simulink model "Simulation_StateLinear_PostureReg"  (R2022b)
settings: Solver=FixedStepAuto  StartTime=0.0  StopTime=200  FixedStep=0.02  RelTol=1e-3
undefined symbols (not defined in the file): theta_des, theta_f, unicycle, x_des, x_f, y_des, y_f
libraries: simulink_extras x3, dspsigops x2
settings Model: Creator=Musta  LastModifiedBy=Musta

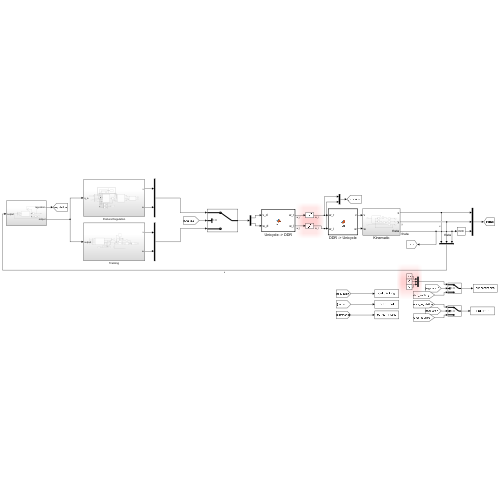
[thumbnail: Simulink's stored preview of the top-level diagram]
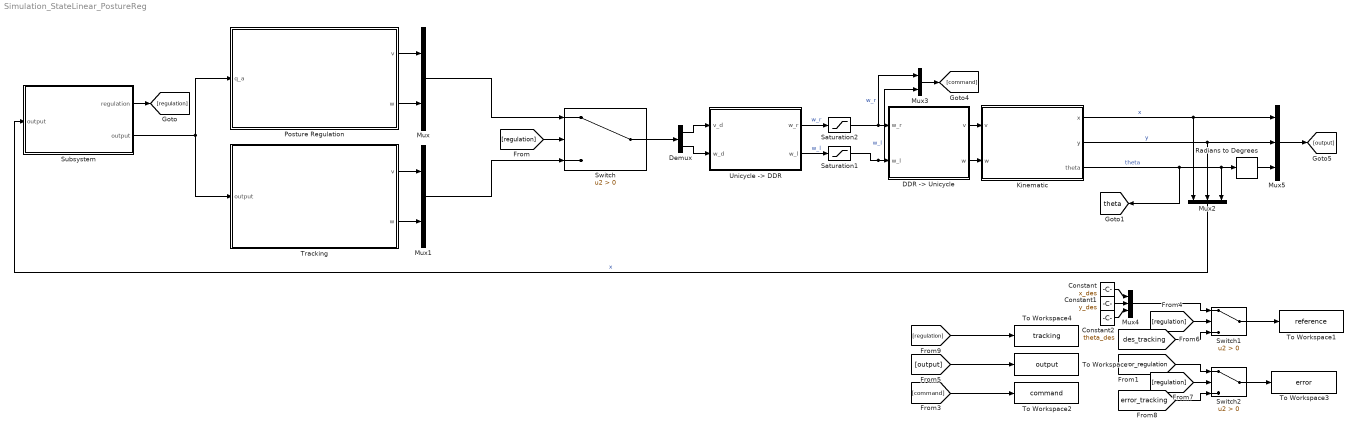
== system Simulation_StateLinear_PostureReg ==
  " DDR -> Unicycle " : MATLAB Function  TreatAsAtomicUnit=on
  Constant : Constant  Value=x_des
  Constant1 : Constant  Value=y_des
  Constant2 : Constant  Value=theta_des
  Demux : Demux  Outputs=2
  Kinematic : Subsystem
  Mux : Mux  Inputs=2
  Mux1 : Mux  Inputs=2
  Mux2 : Mux  Inputs=3
  Mux3 : Mux  Inputs=2
  Mux4 : Mux  Inputs=3
  Mux5 : Mux  Inputs=3
  Posture Regulation : Subsystem
  Radians to Degrees : simulink_extras/Transformations/Radians to Degrees
  Saturation1 : Saturate  UpperLimit=unicycle.omegaWheelMax  LowerLimit=unicycle.omegaWheelMin
  Saturation2 : Saturate  UpperLimit=unicycle.omegaWheelMax  LowerLimit=unicycle.omegaWheelMin
  Subsystem : Subsystem
  Switch : Switch  Criteria=u2 > Threshold  SaturateOnIntegerOverflow=off  InputSameDT=off
  Switch1 : Switch  Criteria=u2 > Threshold  SaturateOnIntegerOverflow=off  InputSameDT=off
  Switch2 : Switch  Criteria=u2 > Threshold  SaturateOnIntegerOverflow=off  InputSameDT=off
  To Workspace : ToWorkspace  VariableName=output  SaveFormat=Structure With Time  SampleTime=-1
  To Workspace1 : ToWorkspace  VariableName=reference  SaveFormat=Structure With Time  SampleTime=-1
  To Workspace2 : ToWorkspace  VariableName=command  SaveFormat=Structure With Time  SampleTime=-1
  To Workspace3 : ToWorkspace  VariableName=error  SaveFormat=Structure With Time  SampleTime=-1
  To Workspace4 : ToWorkspace  VariableName=tracking  SaveFormat=Structure With Time  SampleTime=-1
  Tracking : Subsystem
  "Unicycle -> DDR" : MATLAB Function  TreatAsAtomicUnit=on
  tag scope: theta=global
  wires:
  [error_regulation] -> Switch2/1
  [regulation] -> Switch2/2
  Switch1/1 -> To Workspace1/1
  Subsystem/2(output) -> Posture Regulation/1(q_a), Tracking/1(output)
  Switch/1 -> Demux/1
  Mux1/1 -> Switch/3
  Tracking/2(w) -> Mux1/2
  Mux2/1 -> Subsystem/1("output ")  "x"
  [regulation] -> Switch/2
  [command] -> To Workspace2/1
  Posture Regulation/2(w) -> Mux/2
  Subsystem/1(regulation) -> [regulation]
  [error_tracking] -> Switch2/3
  Saturation1/1 -> Mux3/2, " DDR -> Unicycle "/2(w_l)  "w_l"
  "Unicycle -> DDR"/2(w_l) -> Saturation1/1  "w_l"
  Demux/1 -> "Unicycle -> DDR"/1(v_d)
  Posture Regulation/1(v) -> Mux/1
  Tracking/1(v) -> Mux1/1
  Mux/1 -> Switch/1
  [output] -> To Workspace/1
  Saturation2/1 -> Mux3/1, " DDR -> Unicycle "/1(w_r)  "w_r"
  Switch2/1 -> To Workspace3/1
  "Unicycle -> DDR"/1(w_r) -> Saturation2/1  "w_r"
  Demux/2 -> "Unicycle -> DDR"/2(w_d)
  Kinematic/2(y) -> Mux2/2, Mux5/2  "y"
  " DDR -> Unicycle "/1(v) -> Kinematic/1(v)
  Radians to Degrees/1 -> Mux5/3
  " DDR -> Unicycle "/2(w) -> Kinematic/2(w)
  Mux5/1 -> [output]
  Kinematic/3(theta) -> [theta], Mux2/3, Radians to Degrees/1  "theta"
  Kinematic/1(x) -> Mux2/1, Mux5/1  "x"
  Mux3/1 -> [command]
  [regulation] -> To Workspace4/1
  Mux4/1 -> Switch1/1
  [regulation] -> Switch1/2
  [des_tracking] -> Switch1/3
  Constant1/1 -> Mux4/2
  Constant/1 -> Mux4/1
  Constant2/1 -> Mux4/3

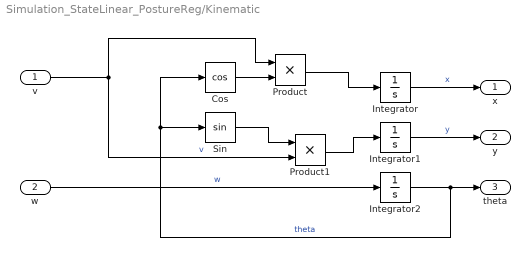
== system Simulation_StateLinear_PostureReg/Kinematic ==
  v : Inport
  w : Inport  Port=2
  Cos : Trigonometry  Operator=cos
  Integrator : Integrator  InitialCondition=unicycle.ic.x
  Integrator1 : Integrator  InitialCondition=unicycle.ic.y
  Integrator2 : Integrator  InitialCondition=unicycle.ic.theta
  Product : Product
  Product1 : Product
  Sin : Trigonometry
  x : Outport
  y : Outport  Port=2
  theta : Outport  Port=3
  wires:
  w/1 -> Integrator2/1  "w"
  Product/1 -> Integrator/1
  v/1 -> Product/1, Product1/2  "v"
  Cos/1 -> Product/2
  Integrator1/1 -> y/1  "y"
  Integrator/1 -> x/1  "x"
  Integrator2/1 -> Cos/1, Sin/1, theta/1  "theta"
  Product1/1 -> Integrator1/1
  Sin/1 -> Product1/1

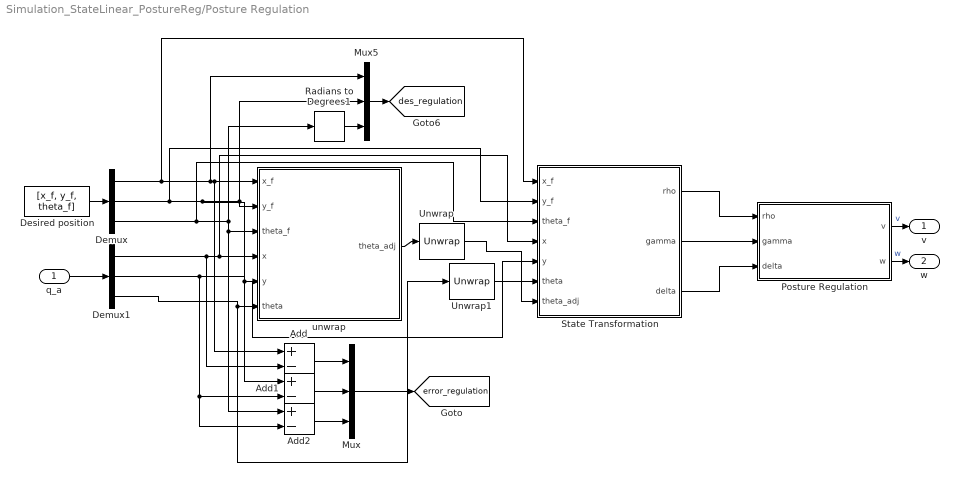
== system Simulation_StateLinear_PostureReg/Posture Regulation ==
  q_a : Inport
  Add : Sum  Inputs=+-
  Add1 : Sum  Inputs=+-
  Add2 : Sum  Inputs=+-
  Demux : Demux  Outputs=3
  Demux1 : Demux  Outputs=3
  Desired position : Constant  Value=[x_f, y_f, theta_f]
  Mux : Mux  Inputs=3
  Mux5 : Mux  Inputs=3
  Posture Regulation : MATLAB Function  TreatAsAtomicUnit=on
  Radians to Degrees1 : simulink_extras/Transformations/Radians to Degrees
  State Transformation : MATLAB Function  TreatAsAtomicUnit=on
  Unwrap : dspsigops/Unwrap  tol=pi  InputProcessing=Columns as channels (frame based)  running=off
  Unwrap1 : dspsigops/Unwrap  tol=pi  InputProcessing=Columns as channels (frame based)  running=off
  unwrap : MATLAB Function  TreatAsAtomicUnit=on
  v : Outport
  w : Outport  Port=2
  tag scope: des_regulation=global, error_regulation=global
  wires:
  Posture Regulation/1(v) -> v/1  "v"
  Radians to Degrees1/1 -> Mux5/3
  Posture Regulation/2(w) -> w/1  "w"
  Mux5/1 -> [des_regulation]
  Desired position/1 -> Demux/1
  Demux/3 -> State Transformation/3(theta_f), Add2/1, unwrap/3(theta_f), Radians to Degrees1/1
  Demux/2 -> State Transformation/2(y_f), Add1/1, Mux5/2, unwrap/2(y_f)
  Demux/1 -> State Transformation/1(x_f), Mux5/1, Add/1, unwrap/1(x_f)
  Demux1/1 -> Add/2, State Transformation/4(x), unwrap/4(x)
  Demux1/2 -> Add2/2, Add1/2, State Transformation/5(y), unwrap/5(y)
  Demux1/3 -> Unwrap1/1, unwrap/6(theta)
  q_a/1 -> Demux1/1
  Add/1 -> Mux/1
  Add1/1 -> Mux/2
  Add2/1 -> Mux/3
  Mux/1 -> [error_regulation]
  State Transformation/2(gamma) -> Posture Regulation/2(gamma)
  State Transformation/1(rho) -> Posture Regulation/1(rho)
  State Transformation/3(delta) -> Posture Regulation/3(delta)
  unwrap/1(theta_adj) -> Unwrap/1
  Unwrap/1 -> State Transformation/7(theta_adj)
  Unwrap1/1 -> State Transformation/6(theta)

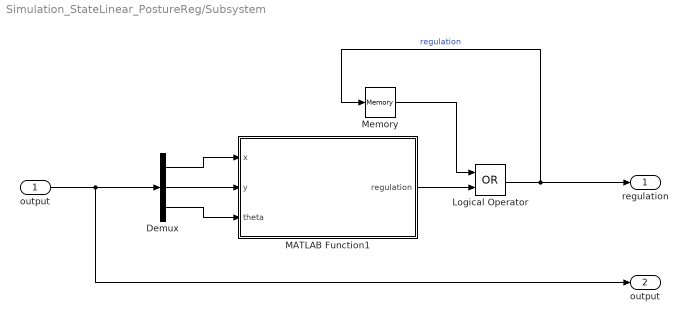
== system Simulation_StateLinear_PostureReg/Subsystem ==
  "output " : Inport
  Demux : Demux  Outputs=3
  Logical Operator : Logic  Operator=OR  AllPortsSameDT=off  OutDataTypeStr=boolean
  MATLAB Function1 : MATLAB Function  TreatAsAtomicUnit=on
  Memory : Memory
  regulation : Outport
  output : Outport  Port=2
  wires:
  Memory/1 -> Logical Operator/1
  Logical Operator/1 -> regulation/1, Memory/1  "regulation"
  MATLAB Function1/1(regulation) -> Logical Operator/2
  "output "/1 -> output/1, Demux/1
  Demux/3 -> MATLAB Function1/3(theta)
  Demux/2 -> MATLAB Function1/2(y)
  Demux/1 -> MATLAB Function1/1(x)

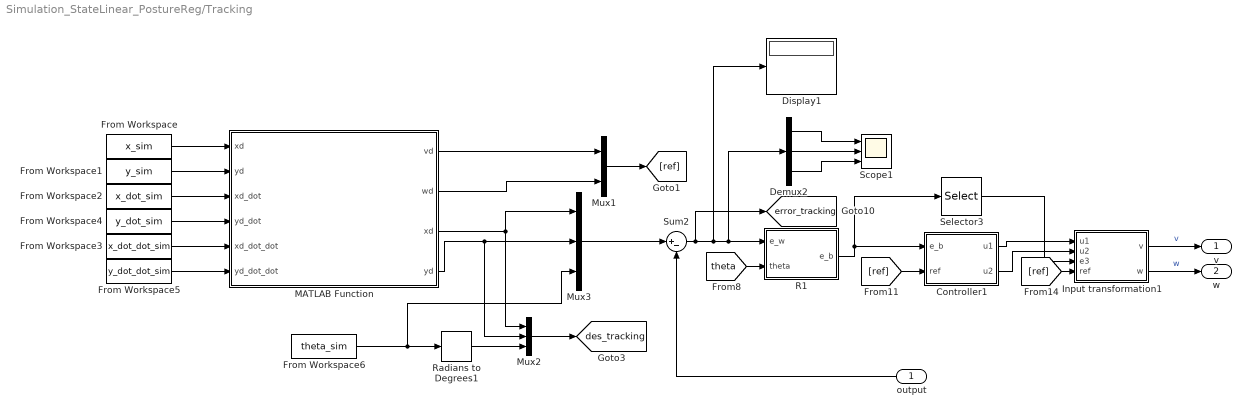
== system Simulation_StateLinear_PostureReg/Tracking ==
  output : Inport
  Controller1 : MATLAB Function  TreatAsAtomicUnit=on
  Demux2 : Demux  Outputs=3
  Display1 : Display
  From Workspace : FromWorkspace  VariableName=x_sim
  From Workspace1 : FromWorkspace  VariableName=y_sim
  From Workspace2 : FromWorkspace  VariableName=x_dot_sim
  From Workspace3 : FromWorkspace  VariableName=x_dot_dot_sim
  From Workspace4 : FromWorkspace  VariableName=y_dot_sim
  From Workspace5 : FromWorkspace  VariableName=y_dot_dot_sim
  From Workspace6 : FromWorkspace  VariableName=theta_sim
  Input transformation1 : MATLAB Function  TreatAsAtomicUnit=on
  MATLAB Function : MATLAB Function  TreatAsAtomicUnit=on
  Mux1 : Mux  Inputs=2
  Mux2 : Mux  Inputs=3
  Mux3 : Mux  Inputs=3
  R1 : MATLAB Function  TreatAsAtomicUnit=on
  Radians to Degrees1 : simulink_extras/Transformations/Radians to Degrees
  Scope1 : Scope  NumInputPorts=3
  Selector3 : Selector  InputPortWidth=3  IndexOptions=Index vector (dialog)  Indices=3  OutputSizes=1
  Sum2 : Sum  Inputs=|+-
  v : Outport
  w : Outport  Port=2
  tag scope: des_tracking=global, error_tracking=global
  wires:
  Sum2/1 -> [error_tracking], Display1/1, R1/1(e_w), Demux2/1
  [theta] -> R1/2(theta)
  Input transformation1/1(v) -> v/1  "v"
  Selector3/1 -> Input transformation1/3(e3)
  Demux2/2 -> Scope1/2
  R1/1(e_b) -> Selector3/1, Controller1/1(e_b)
  Controller1/1(u1) -> Input transformation1/1(u1)
  Demux2/1 -> Scope1/1
  [ref] -> Controller1/2(ref)
  [ref] -> Input transformation1/4(ref)
  Demux2/3 -> Scope1/3
  Controller1/2(u2) -> Input transformation1/2(u2)
  output/1 -> Sum2/2
  Input transformation1/2(w) -> w/1  "w"
  Radians to Degrees1/1 -> Mux2/3
  From Workspace5/1 -> MATLAB Function/6(yd_dot_dot)
  From Workspace1/1 -> MATLAB Function/2("yd ")
  MATLAB Function/1(vd) -> Mux1/1
  Mux1/1 -> [ref]
  From Workspace3/1 -> MATLAB Function/5(xd_dot_dot)
  MATLAB Function/3(xd) -> Mux3/1, Mux2/1
  From Workspace/1 -> MATLAB Function/1("xd ")
  MATLAB Function/2(wd) -> Mux1/2
  From Workspace4/1 -> MATLAB Function/4(yd_dot)
  MATLAB Function/4(yd) -> Mux2/2, Mux3/2
  Mux2/1 -> [des_tracking]
  From Workspace6/1 -> Radians to Degrees1/1, Mux3/3
  From Workspace2/1 -> MATLAB Function/3(xd_dot)
  Mux3/1 -> Sum2/1

== matlab function Simulation_StateLinear_PostureReg/Unicycle -> DDR ==
  data: v_d input; w_r output; w_d input; w_l output
function [w_r, w_l] = fcn(v_d, w_d)

    %#codegen
    coder.extrinsic('evalin')
    d = 0;                  % Needed in order to set variable class correctly
    r = 0;                  % Needed in order to set variable class correctly
    d = evalin('base','unicycle.d'); % Read value from workspace
    r = evalin('base','unicycle.r'); % Read value from workspace

    w_r = ((2 * v_d) + (w_d * d)) / (2 * r);
    w_l = ((2 * v_d) - (w_d * d)) / (2 * r);

end

== matlab function Simulation_StateLinear_PostureReg/Subsystem/MATLAB Function1 ==
  data: x input; regulation output; y input; theta input
function regulation = fcn(x,y,theta)

    coder.extrinsic('evalin')
    x_des = 0;                  % Needed in order to set variable class correctly
    y_des = 0;                  % Needed in order to set variable class correctly
    x_des = evalin('base','x_des'); % Read value from workspace
    y_des = evalin('base','y_des'); % Read value from workspace

    th = 0.01;

    if (abs(x)<abs(x_des)+th) && (abs(x)>abs(x_des)-th) && (abs(y)<abs(y_des)+th) && (abs(y)>abs(y_des)-th)
        regulation = 1;
    else
        regulation = 0;
    end

end

== matlab function Simulation_StateLinear_PostureReg/Posture Regulation/Posture Regulation ==
  data: v output; w output; rho input; gamma input; delta input
function [v,w] = fcn(rho,gamma,delta)

    %#codegen
    coder.extrinsic('evalin')
    k1 = 0;                  % Needed in order to set variable class correctly
    k2 = 0;                  % Needed in order to set variable class correctly
    k3 = 0;                  % Needed in order to set variable class correctly
    k1 = evalin('base','k1'); % Read value from workspace
    k2 = evalin('base','k2'); % Read value from workspace
    k3 = evalin('base','k3'); % Read value from workspace

    v = k1 * rho * cos(gamma);
    w = k2 * gamma + k1 *(sin(gamma)*cos(gamma))*(gamma + k3 * delta)/gamma;

    if rho < 10^-1
        v = .05*v;
        w = .05*w;
        if rho < .01 && abs(gamma) < deg2rad(1) && abs(delta) <  deg2rad(1)
            v = 0.0;
            w = 0.0;
        elseif rho < .025 && abs(gamma) < deg2rad(5) && abs(delta) <  deg2rad(5)
            v = .015*v;
            w = .015*w;
        elseif rho < .05 && abs(gamma) < deg2rad(10) && abs(delta) <  deg2rad(10)
            v = .03*v;
            w = .03*w;
        end 
    end 

end

== matlab function Simulation_StateLinear_PostureReg/Tracking/MATLAB Function ==
  data: xd input; vd output; yd input; xd_dot input; yd_dot input; xd_dot_dot input; yd_dot_dot input; wd output; xd output; yd output
function [vd, wd, xd, yd] = fcn(xd, yd, xd_dot, yd_dot, xd_dot_dot, yd_dot_dot)
    
    vd = sqrt(xd_dot.^2 + yd_dot.^2);
    wd = (xd_dot.*yd_dot_dot - xd_dot_dot.*yd_dot) / (xd_dot.^2 + yd_dot.^2);

    xd = xd;
    yd = yd;

end

== matlab function Simulation_StateLinear_PostureReg/Posture Regulation/unwrap ==
  data: x_f input; theta_adj output; y_f input; theta_f input; x input; y input; theta input
function theta_adj = fcn(x_f, y_f, theta_f, x, y, theta)

    e_x = x_f - x;
    e_y = y_f - y;
    e_theta = theta_f - theta;
   
    theta_adj = atan2(e_y,e_x);

end

== matlab function Simulation_StateLinear_PostureReg/ DDR -> Unicycle  ==
  data: w_r input; v output; w_l input; w output
function [v, w] = fcn(w_r, w_l)

    %#codegen
    coder.extrinsic('evalin')
    d = 0;                  % Needed in order to set variable class correctly
    r = 0;                  % Needed in order to set variable class correctly
    d = evalin('base','unicycle.d'); % Read value from workspace
    r = evalin('base','unicycle.r'); % Read value from workspace

    v = r*(w_r + w_l)/2; % rad/s
    w = r*(w_r - w_l)/d; % rad/s

end

== matlab function Simulation_StateLinear_PostureReg/Tracking/Controller1 ==
  data: e_b input; u1 output; ref input; u2 output
function [u1,u2] = fcn(e_b, ref)

    %#codegen
    coder.extrinsic('evalin')
    a = 0;                  % Needed in order to set variable class correctly
    zeta = 0;                  % Needed in order to set variable class correctly
    a = evalin('base','a'); % Read value from workspace
    zeta = evalin('base','zeta'); % Read value from workspace

    k1 = 2*zeta*a;
    k2 = (a^2 - ref(2)^2) / ref(1);
    k3 = 2*zeta*a;

    u1 = -k1*e_b(1);
    u2 = -k2*e_b(2) -k3*e_b(3);

end

== matlab function Simulation_StateLinear_PostureReg/Tracking/Input transformation1 ==
  data: u1 input; v output; u2 input; e3 input; w output; ref input
function [v, w] = fcn(u1, u2, e3, ref)

    v = ref(1)*cos(e3) - u1;
    w = ref(2) - u2;

end

== matlab function Simulation_StateLinear_PostureReg/Posture Regulation/State Transformation ==
  data: x_f input; rho output; y_f input; gamma output; delta output; theta_f input; x input; y input; theta input; theta_adj input
function [rho,gamma,delta] = fcn(x_f, y_f, theta_f, x, y, theta, theta_adj)

    e_x = x_f - x;
    e_y = y_f - y;
    e_theta = theta_f - theta;
   
    rho = sqrt(e_x^2 + e_y^2);
    gamma = theta_adj - theta;
    delta = gamma - e_theta;

end

== matlab function Simulation_StateLinear_PostureReg/Tracking/R1 ==
  data: e_w input; e_b output; theta input
function e_b  = fcn(e_w, theta)
    
    R = [cos(theta), sin(theta), 0;
        -sin(theta), cos(theta), 0;
         0, 0, 1];

    e_b = R * e_w;

end
